simulink model "Product1"  (R2017b)
settings: Solver=FixedStepDiscrete  StartTime=0.0  StopTime=10.0  FixedStep=0.200000  RelTol=1e-3  EnableMultiTasking=on
model workspace (MAT data in the model file):
  already_pp = 0
  input_struct.time = [0; 0.2; 0.4; 0.6; 0.8; 1; 1.2; 1.4; 1.6; 1.8; 2; 2.2; 2.4; 2.6; 2.8; 3; 3.2; 3.4; 3.6; 3.8; 4; 4.2; 4.4; 4.6; 4.8; 5; 5.2; 5.4; 5.6; 5.8; 6; 6.2; 6.4; 6.6; 6.8; 7; 7.2; 7.4; 7.6; 7.8; 8; 8.2; 8.4; 8.6; 8.8; 9; 9.2; 9.4; 9.6; 9.8; 10; 10.2; 10.4; 10.6; 10.8; 11; 11.2; 11.4; 11.6; 11.8; 12; 12.2; 12.4; 12.6; 12.8; 13; 13.2; 13.4; 13.6; 13.8; 14; 14.2; 14.4; 14.6; 14.8; 15; 15.2; 15.4; 15.6; 15.8; 16; 16.2; 16.4; 16.6; 16.8; 17; 17.2; 17.4; 17.6; 17.8; 18; 18.2; 18.4; 18.6; 18.8; 19; 19.2; 19.4; 19.6; 19.8]
  input_struct.signals(1).name = 'In1'
  input_struct.signals(1).values = [30.0718881487 -21.6360189193 43.6528842244 76.2732413054 -97.4592547622 -85.3131272562 -23.5122204412 34.0367023267 99.1051504353 10.1175948133 16.5590594005 -45.0133750219 ... (600 elements, 2x3x100)]
  input_struct.signals(1).dimensions = [2 3]
  input_struct.signals(2).name = 'In2'
  input_struct.signals(2).values = [43.3795484024 99.1638979857 27.8435485869 0.493874764616 8.66581062646 -53.8386882301 33.7043671481 1.23460647022 14.568842137 -95.7712771188 46.4868819004 21.740169656 ... (600 elements, 3x2x100)]
  input_struct.signals(2).dimensions = [3 2]
settings Model: Creator=hbourbou  LastModifiedBy=hbourbou
settings DataIOCC: SaveFormat=StructureWithTime
settings OptimizationCC: LifeSpan=inf
settings DebuggingCC: AlgebraicLoopMsg=error  ArtificialAlgebraicLoopMsg=error  SFExecutionAtInitializationDiag=none
settings HardwareCC: ProdBitPerSizeT=32  ProdBitPerPtrDiffT=32  ProdWordSize=32  ProdHWDeviceType=Specified
settings CodeAppCC: StateflowObjectComments=on

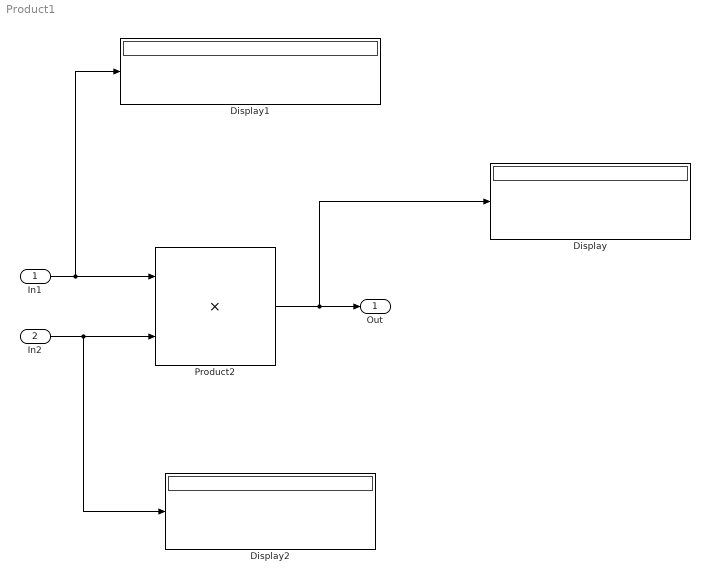
== system Product1 ==
  In1 : Inport  OutDataTypeStr=double  PortDimensions=[3 2]
  In2 : Inport  Port=2  OutDataTypeStr=double  PortDimensions=[3 2]
  Display : Display
  Display1 : Display
  Display2 : Display
  Product2 : Product
  Out : Outport
  wires:
  In1/1 -> Display1/1, Product2/1
  In2/1 -> Display2/1, Product2/2
  Product2/1 -> Display/1, Out/1
